simulink model "Part2_4"  (R2018a)
settings: Solver=FixedStepDiscrete  StartTime=0.0  StopTime=3  FixedStep=10e-6  MaxStep=0.2  RelTol=1e-4
libraries: powerlib x11
settings Model: Creator=Batuhan  LastModifiedBy=Batuhan
settings CodeAppCC: StateflowObjectComments=on

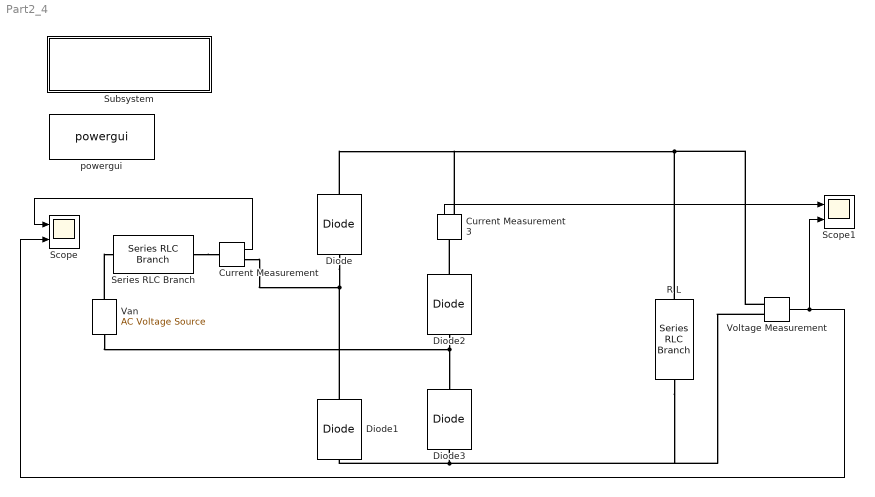
== system Part2_4 ==
  Current Measurement : powerlib/Measurements/Current Measurement  PhasorSimulation=off  OutputType=Complex  PSBequivalent=0
  Current Measurement3 : powerlib/Measurements/Current Measurement  PhasorSimulation=off  OutputType=Complex  PSBequivalent=0
  Diode{,1..3} (4 alike) : powerlib/Power Electronics/Diode  Ron=0.001  Lon=0  Vf=0.8  IC=0  UseSnubber=0  Rs=1e5  Cs=inf  Measurements=off
  R L : powerlib/Elements/Series RLC Branch  LConnTagsString=__new0  RConnTagsString=__new0  BranchType=RL  Resistance=100  Inductance=1  SetiL0=off  InitialCurrent=0  Capacitance=470e-9  Setx0=off  InitialVoltage=0  Measurements=None
  Scope : Scope  NumInputPorts=2
  Scope1 : Scope  NumInputPorts=2
  Series RLC Branch : powerlib/Elements/Series RLC Branch  LConnTagsString=__new0  RConnTagsString=__new0  BranchType=L  Resistance=1  Inductance=10e-3  SetiL0=off  InitialCurrent=0  Capacitance=1e-6  Setx0=off  InitialVoltage=0  Measurements=None
  Subsystem : Subsystem
      settings: OpenFcn=open_system('power_new_palette')
      mask Display: disp(sprintf('Open Simscape Power Systems\n(Specialized Technology)\nPalette Library'));
  Van : powerlib/Electrical Sources/AC Voltage Source  Amplitude=325.27  Phase=0  Frequency=50  SampleTime=0  Measurements=None  BusType=swing  Pref=10e3  Qref=0  Qmin=-inf  Qmax=+inf
  Voltage Measurement : powerlib/Measurements/Voltage Measurement  PhasorSimulation=off  OutputType=Complex  PSBequivalent=0
  powergui : powerlib/powergui  Priority=1  SimulationMode=Discrete  SampleTime=10e-6  frequency=60  Iterations=50  frequencyindice=50  Pbase=100e6  ErrMax=1e-4  UnitsV=kV  UnitsW=MW  buscounter=0  FunctionMessages=off  echomessages=off  EnableUseOfTLC=off  CurrentSourceSwitches=off  DisableSnubberDevices=off  DisableRonSwitches=off  DisableVfSwitches=off  DisplayEquations=off  SolverType=Tustin/Backward Euler (TBE)  Interpol=off  ExternalGateDelay=off  methode=off  Ts=100  x0status=blocks  SPID=off  SwTol=0  HookPort=off  RestoreLinks=warning  ResistiveCurrentMeasurement=off  Frange=[0:2:500]  Ylog=off  Xlog=on  ShowGrid=off  save=off  variable=ZData  structure=LineCurrent  ZoomFFT=off  StartTime=0.5  cycles=30  DisplayStyle=1  fundamental=50  FreqAxis=off  MaxFrequency=1000  frequencyindicesteady=1  RmsSteady=2  display=off
  wires:
  Voltage Measurement/1 -> Scope1/2, Scope/2
  Current Measurement/1 -> Scope/1
  Current Measurement3/1 -> Scope1/1
  connections:
  Van/LConn1 -- Diode2/LConn1 -- Diode3/RConn1
  Current Measurement/RConn1 -- Diode1/RConn1 -- Diode/LConn1
  Van/RConn1 -- Series RLC Branch/LConn1
  Voltage Measurement/LConn1 -- Current Measurement3/RConn1 -- Diode/RConn1 -- R L/LConn1
  R L/RConn1 -- Voltage Measurement/LConn2 -- Diode1/LConn1 -- Diode3/LConn1
  Diode2/RConn1 -- Current Measurement3/LConn1
  Series RLC Branch/RConn1 -- Current Measurement/LConn1

== system Part2_4/Subsystem ==
